simulink model "SGP_estimator"  (Simulink 7.4)
settings: Solver=ode4  StartTime=0.0  StopTime=120000  FixedStep=s_FRAME_SIZE  RelTol=1e-3
values from neighbouring files (symbols this model uses):
  equinox = datenum('21-Mar-2010 12:0:0')    [constants_v13.m]    (also in constants_v15.m; constants_v15_Pow.m; constants_v15_Pow_ss_error.m; constants_v16_integral_kartavya.m)
  s_FRAME_SIZE = 2    [constants_v13.m]    (also in constants_v15.m; constants_v15_Pow.m; constants_v15_Pow_ss_error.m; constants_v16_integral_kartavya.m)
  stperut = 1.00273790935    [constants_v16_integral_kartavya.m]    (also in constants_v16_integral_light_sun_sgp_igrf_power_13Dec2011.m; precalcs.m)
  t_reset = 600    [constants_v16_integral_kartavya.m]    (also in constants_v16_integral_light_sun_sgp_igrf_power_13Dec2011.m; precalcs.m)
  today = datenum('18-Oct-2010 10:30:0')    [constants_v13.m]    (also in constants_v15.m; constants_v15_Pow.m; constants_v15_Pow_ss_error.m; constants_v16_integral_kartavya.m)
  W_EARTH_ROT = 2*pi/86400    (= 7.27220521664e-05)    [constants_v16_integral_kartavya.m]    (also in constants_v16_integral_light_sun_sgp_igrf_power_13Dec2011.m; precalcs.m)
libraries: commnoisgen2 x2, aerolibutil x1
settings Model: Creator=Jaideep  LastModifiedBy=Jaideep
settings SolverCC: AutoInsertRateTranBlk=on

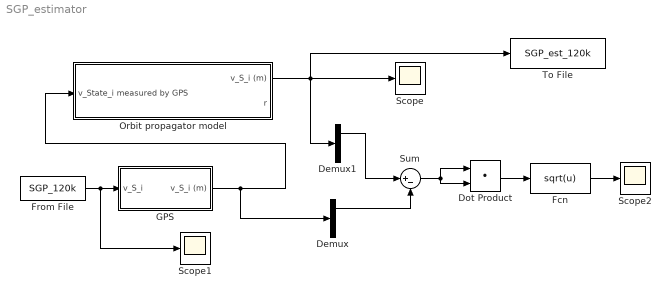
== system SGP_estimator ==
  Demux : Demux  Outputs=2
  Demux1 : Demux  Outputs=2
  Dot Product : DotProduct  OutDataType=fixdt(1, 16)  OutScaling=2^-10  InputSameDT=on  OutDataTypeStr=Inherit: Inherit via internal rule
  Fcn : Fcn  Expr=sqrt(u)
  From File : FromFile  FileName=SGP_120k  SampleTime=0
  GPS : Subsystem
  Orbit propagator model : Subsystem
  Scope : Scope
      settings: YMin=-4e+006  YMax=8e+006
  Scope1 : Scope
  Scope2 : Scope
      settings: YMin=50000  YMax=575000  SaveName=ScopeData2
  Sum : Sum  Inputs=|+-  OutDataType=fixdt(1, 16)  OutScaling=2^0
  To File : ToFile  Filename=SGP_est_120k  MatrixName=SGP_est_120k
  wires:
  GPS/1(v_S_i (m)) -> Orbit propagator model/1(v_State_i measured by GPS), Demux/1
  From File/1 -> GPS/1(v_S_i), Scope1/1
  Orbit propagator model/1(v_S_i (m)) -> Demux1/1, Scope/1, To File/1
  Demux1/1 -> Sum/1
  Demux/1 -> Sum/2
  Sum/1 -> Dot Product/1, Dot Product/2
  Dot Product/1 -> Fcn/1
  Fcn/1 -> Scope2/1

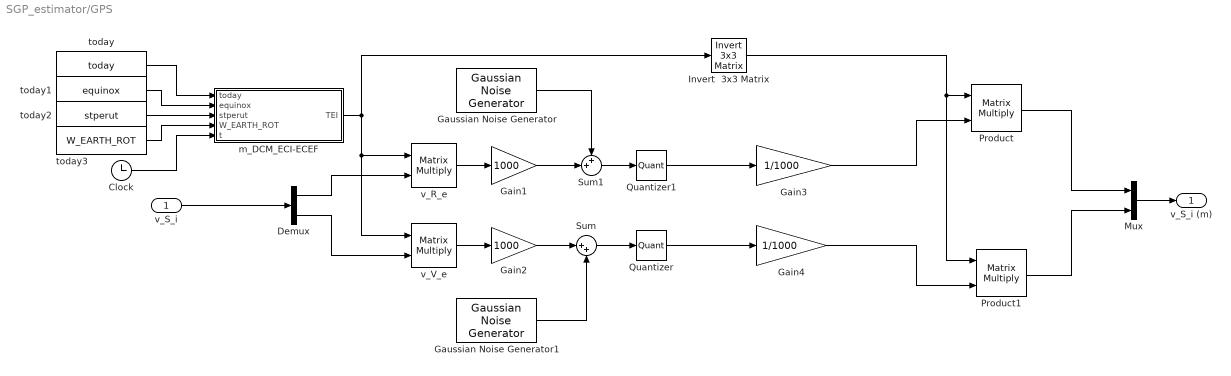
== system SGP_estimator/GPS ==
  v_S_i : Inport  OutDataType=sfix(16)  OutScaling=2^0
  Clock : Clock
      settings: Decimation=10
  Demux : Demux  Outputs=2
  Gain1 : Gain  Gain=1000  ParameterDataType=sfix(16)  ParameterScaling=2^0  OutDataType=sfix(16)  OutScaling=2^0
  Gain2 : Gain  Gain=1000  ParameterDataType=sfix(16)  ParameterScaling=2^0  OutDataType=sfix(16)  OutScaling=2^0
  Gain3 : Gain  Gain=1/1000  ParameterDataType=sfix(16)  ParameterScaling=2^0  OutDataType=sfix(16)  OutScaling=2^0
  Gain4 : Gain  Gain=1/1000  ParameterDataType=sfix(16)  ParameterScaling=2^0  OutDataType=sfix(16)  OutScaling=2^0
  Gaussian Noise Generator : commnoisgen2/Gaussian Noise Generator  SystemSampleTime=-1  m=0  d=s_x_GPS_X  s=41  Ts=s_FRAME_SIZE  frameBased=off  sampPerFrame=1  orient=off  outDataType=double
  Gaussian Noise Generator1 : commnoisgen2/Gaussian Noise Generator  SystemSampleTime=-1  m=0  d=s_x_GPS_V  s=24  Ts=s_FRAME_SIZE  frameBased=off  sampPerFrame=1  orient=off  outDataType=double
  Invert  3x3 Matrix : aerolibutil/Invert  3x3 Matrix  SystemSampleTime=-1
  Mux : Mux  Inputs=2
  Product : Product  Multiplication=Matrix(*)  OutDataType=sfix(16)  OutScaling=2^0  RndMeth=Zero
  Product1 : Product  Multiplication=Matrix(*)  OutDataType=sfix(16)  OutScaling=2^0  RndMeth=Zero
  Quantizer : Quantizer  QuantizationInterval=1/(2^31)
  Quantizer1 : Quantizer  QuantizationInterval=1/(2^31)
  Sum : Sum  Inputs=|++  OutDataType=sfix(16)  OutScaling=2^0
  Sum1 : Sum  Inputs=++|  OutDataType=sfix(16)  OutScaling=2^0
  m_DCM_ECI-ECEF : Stateflow chart
  today : Constant  Value=today  OutDataType=sfix(16)  OutScaling=2^0
  today1 : Constant  Value=equinox  OutDataType=sfix(16)  OutScaling=2^0
  today2 : Constant  Value=stperut  OutDataType=sfix(16)  OutScaling=2^0
  today3 : Constant  Value=W_EARTH_ROT  OutDataType=sfix(16)  OutScaling=2^0
  v_R_e : Product  Multiplication=Matrix(*)  OutDataType=sfix(16)  OutScaling=2^0  RndMeth=Zero
  v_V_e : Product  Multiplication=Matrix(*)  OutDataType=sfix(16)  OutScaling=2^0  RndMeth=Zero
  v_S_i (m) : Outport  OutDataType=sfix(16)  OutScaling=2^0
  wires:
  Gaussian Noise Generator/1 -> Sum1/1
  Gaussian Noise Generator1/1 -> Sum/2
  Product1/1 -> Mux/2
  Gain4/1 -> Product1/2
  Product/1 -> Mux/1
  Gain3/1 -> Product/2
  Invert  3x3 Matrix/1 -> Product1/1, Product/1
  Quantizer1/1 -> Gain3/1
  Mux/1 -> v_S_i (m)/1
  Sum/1 -> Quantizer/1
  Sum1/1 -> Quantizer1/1
  Gain1/1 -> Sum1/2
  Gain2/1 -> Sum/1
  v_R_e/1 -> Gain1/1
  v_V_e/1 -> Gain2/1
  Quantizer/1 -> Gain4/1
  Clock/1 -> m_DCM_ECI-ECEF/5(t)
  Demux/2 -> v_V_e/2
  Demux/1 -> v_R_e/2
  v_S_i/1 -> Demux/1
  today3/1 -> m_DCM_ECI-ECEF/4(W_EARTH_ROT)
  today2/1 -> m_DCM_ECI-ECEF/3(stperut)
  today1/1 -> m_DCM_ECI-ECEF/2(equinox)
  today/1 -> m_DCM_ECI-ECEF/1(today)
  m_DCM_ECI-ECEF/1(TEI) -> Invert  3x3 Matrix/1, v_V_e/1, v_R_e/1

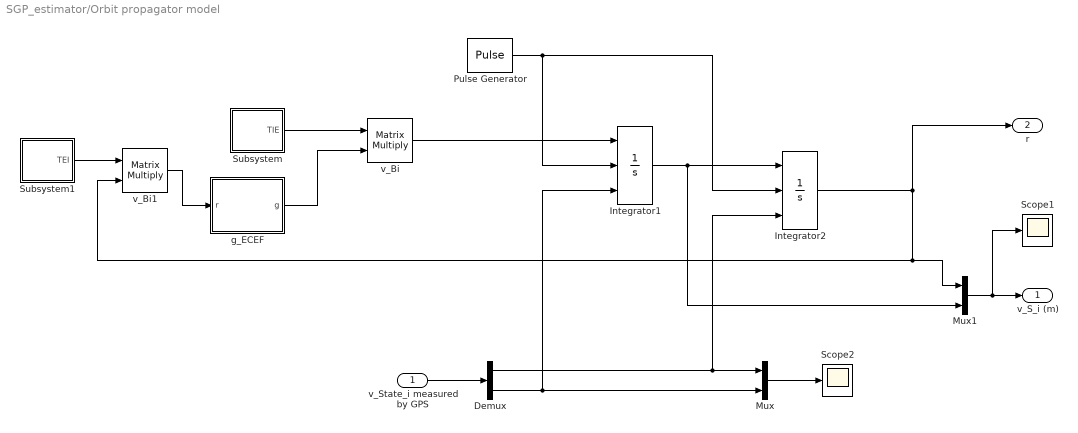
== system SGP_estimator/Orbit propagator model ==
  v_State_i measured by GPS : Inport
  Demux : Demux  Outputs=2
  Integrator1 : Integrator  ExternalReset=rising  InitialConditionSource=external
  Integrator2 : Integrator  ExternalReset=rising  InitialConditionSource=external
  Mux : Mux  Inputs=2
  Mux1 : Mux  Inputs=2
  Pulse Generator : DiscretePulseGenerator  PulseType=Time based  Amplitude=1  Period=t_reset  PulseWidth=50  PhaseDelay=0  SampleTime=1
  Scope1 : Scope
      settings: SaveName=ScopeData26  SampleInput=on
  Scope2 : Scope
      settings: SaveName=ScopeData4  SampleInput=on
  Subsystem : Subsystem
  Subsystem1 : Subsystem
  g_ECEF : Stateflow chart
  v_Bi : Product  Multiplication=Matrix(*)  OutDataType=sfix(16)  OutScaling=2^0  RndMeth=Zero
  v_Bi1 : Product  Multiplication=Matrix(*)  OutDataType=sfix(16)  OutScaling=2^0  RndMeth=Zero
  v_S_i (m) : Outport  OutDataType=sfix(16)  OutScaling=2^0
  r : Outport  Port=2  OutDataType=sfix(16)  OutScaling=2^0
  wires:
  Pulse Generator/1 -> Integrator1/2, Integrator2/2
  Mux/1 -> Scope2/1
  v_State_i measured by GPS/1 -> Demux/1
  Demux/1 -> Mux/1, Integrator2/3
  Demux/2 -> Mux/2, Integrator1/3
  Integrator2/1 -> r/1, Mux1/1, v_Bi1/2
  Integrator1/1 -> Integrator2/1, Mux1/2
  Mux1/1 -> v_S_i (m)/1, Scope1/1
  Subsystem/1(TIE) -> v_Bi/1
  g_ECEF/1(g) -> v_Bi/2
  v_Bi/1 -> Integrator1/1
  Subsystem1/1(TEI) -> v_Bi1/1
  v_Bi1/1 -> g_ECEF/1(r)

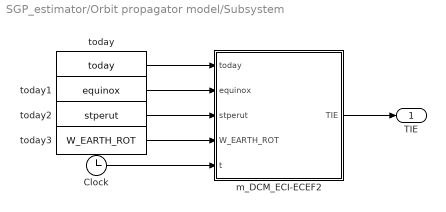
== system SGP_estimator/Orbit propagator model/Subsystem ==
  Clock : Clock
      settings: Decimation=10
  m_DCM_ECI-ECEF2 : Stateflow chart
  today : Constant  Value=today  OutDataType=sfix(16)  OutScaling=2^0
  today1 : Constant  Value=equinox  OutDataType=sfix(16)  OutScaling=2^0
  today2 : Constant  Value=stperut  OutDataType=sfix(16)  OutScaling=2^0
  today3 : Constant  Value=W_EARTH_ROT  OutDataType=sfix(16)  OutScaling=2^0
  TIE : Outport
  wires:
  m_DCM_ECI-ECEF2/1(TIE) -> TIE/1
  Clock/1 -> m_DCM_ECI-ECEF2/5(t)
  today3/1 -> m_DCM_ECI-ECEF2/4(W_EARTH_ROT)
  today2/1 -> m_DCM_ECI-ECEF2/3(stperut)
  today1/1 -> m_DCM_ECI-ECEF2/2(equinox)
  today/1 -> m_DCM_ECI-ECEF2/1(today)

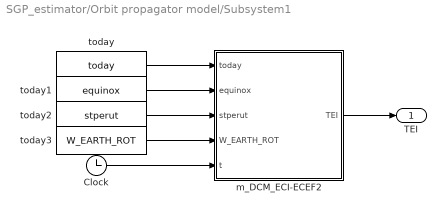
== system SGP_estimator/Orbit propagator model/Subsystem1 ==
  Clock : Clock
      settings: Decimation=10
  m_DCM_ECI-ECEF2 : Stateflow chart
  today : Constant  Value=today  OutDataType=sfix(16)  OutScaling=2^0
  today1 : Constant  Value=equinox  OutDataType=sfix(16)  OutScaling=2^0
  today2 : Constant  Value=stperut  OutDataType=sfix(16)  OutScaling=2^0
  today3 : Constant  Value=W_EARTH_ROT  OutDataType=sfix(16)  OutScaling=2^0
  TEI : Outport
  wires:
  today/1 -> m_DCM_ECI-ECEF2/1(today)
  today1/1 -> m_DCM_ECI-ECEF2/2(equinox)
  today2/1 -> m_DCM_ECI-ECEF2/3(stperut)
  today3/1 -> m_DCM_ECI-ECEF2/4(W_EARTH_ROT)
  Clock/1 -> m_DCM_ECI-ECEF2/5(t)
  m_DCM_ECI-ECEF2/1(TEI) -> TEI/1

== matlab function Orbit propagator model/Subsystem1/m_DCM_ECI-ECEF2 ==
  data: TEI output double; today input double; equinox input double; stperut input double; W_EARTH_ROT input double; t input double
function TEI = fcn(today,equinox, stperut,W_EARTH_ROT,t)
% This block gives DCM for converting from ECI to ECEF frames
% inputs: today's date, equinox, sidereal time per unit time, angular velocity of earth's rotation, simulation time
% output: DCM

% 23hr 56m 4.09s per day

ut_sec = (today - equinox)*24*60*60 + t; % universal time in sec
st_sec = stperut*ut_sec;    % sidereal time in sec

phi = st_sec*W_EARTH_ROT;            % sidereal time in rad

TEI = [ cos(phi) sin(phi) 0;
       -sin(phi) cos(phi) 0;
        0        0        1];

== matlab function Orbit propagator model/g_ECEF ==
  data: r input double; g output double; mu parameter double
function g = fcn(r, mu)
%#eml
R = norm(r);
x = r(1); y= r(2); z = r(3);
a = 6378137;
J2 =  1.08263e-3;
J4 = -1.65597e-6;

% J2 Field
gx = -mu*x/R^3*(1 + 3*J2*a^2/2/R^2 - 15*J2*(a*z)^2/2/R^4);
gy = -mu*y/R^3*(1 + 3*J2*a^2/2/R^2 - 15*J2*(a*z)^2/2/R^4);
gz = -mu*z/R^3*(1 + 9*J2*a^2/2/R^2 - 15*J2*(a*z)^2/2/R^4);

% % J4 field
% gx = -(mu*x*(8*(R^2)^4 + 315*J4*a^4*z^4 + 12*J2*a^2*(R^2)^3 + 15*J4*a^4*(R^2)^2 - 210*J4*a^4*z^2*(R^2) - 60*J2*a^2*z^2*(R^2)^2))/(8*(R^2)^(11/2));
% gy = -(mu*y*(8*(R^2)^4 + 315*J4*a^4*z^4 + 12*J2*a^2*(R^2)^3 + 15*J4*a^4*(R^2)^2 - 210*J4*a^4*z^2*(R^2) - 60*J2*a^2*z^2*(R^2)^2))/(8*(R^2)^(11/2));
% gz = -(mu*z*(8*(R^2)^4 + 315*J4*a^4*z^4 + 36*J2*a^2*(R^2)^3 + 75*J4*a^4*(R^2)^2 - 350*J4*a^4*z^2*(R^2) - 60*J2*a^2*z^2*(R^2)^2))/(8*(R^2)^(11/2));

g = [gx; gy; gz];

== matlab function Orbit propagator model/Subsystem/m_DCM_ECI-ECEF2 ==
  data: TIE output double; today input double; equinox input double; stperut input double; W_EARTH_ROT input double; t input double
function TIE = fcn(today,equinox, stperut,W_EARTH_ROT,t)
% This block gives DCM for converting from ECI to ECEF frames
% inputs: today's date, equinox, sidereal time per unit time, angular velocity of earth's rotation, simulation time
% output: DCM

% 23hr 56m 4.09s per day

ut_sec = (today - equinox)*24*60*60 + t; % universal time in sec
st_sec = stperut*ut_sec;    % sidereal time in sec

phi = st_sec*W_EARTH_ROT;            % sidereal time in rad

TEI = [ cos(phi) sin(phi) 0;
       -sin(phi) cos(phi) 0;
        0        0        1];
TIE = TEI';

== matlab function GPS/m_DCM_ECI-ECEF ==
  data: TEI output double; today input double; equinox input double; stperut input double; W_EARTH_ROT input double; t input double
function TEI = fcn(today,equinox, stperut,W_EARTH_ROT, t)
% This block gives DCM for converting from ECI to ECEF frames
% inputs: today's date, equinox, sidereal time per unit time, angular velocity of earth's rotation, simulation time
% output: DCM

% 23hr 56m 4.09s per day

ut_sec = (today - equinox)*24*60*60 + t; % universal time in sec
st_sec = stperut*ut_sec;    % sidereal time in sec

phi = st_sec*W_EARTH_ROT;            % sidereal time in rad

TEI = [ cos(phi) sin(phi) 0;
       -sin(phi) cos(phi) 0;
        0        0        1];
